simulink library "collection_of_goodies"  (R2018a)
settings: Solver=VariableStepAuto  StartTime=0.0  StopTime=10.0  RelTol=1e-3
undefined symbols (not defined in the file or in its folder): a1_T_CMG, a2_T_CMG, a3_T_CMG, AccLim, b1_T_CMG, b2_T_CMG, b3_T_CMG, c, CFthreshoff, CFthreshon, filt1d, filt1n, filt2d, filt2n, filts1n, filts2d, filts2n, fine, h, h_cos_cmg, h_init, h_sin_cmg, hdmax, hmax, I, I34, Id, Igm1d, Igm1n, IgmAAFd, init, invI, invId, Is, Isat, IsatSp, k1_obs, k2_obs, Kt, Kts, lam, Lgm, ls, lt, M34, Ngear, P0, pfd, pfn, q0, q_init, rc_ampl, rc_harm, rc_phase, Rgm, Smin, SmotDrag, spin_init, TachAAFd, TAU_ACS ... (+9)
libraries: mblibv1 x3, sharedutil x1, dspinverses x1, $bdroot x1
(part 2 of 3)

== system collection_of_goodies/Vector Math/3x3 cross ==
  v : Inport
  Constant1 : Constant  Value=0
  Constant2 : Constant  Value=0
  Constant3 : Constant  Value=0
  Demux : Demux  Outputs=3
  Gain : Gain  Gain=-1  SaturateOnIntegerOverflow=on  OutDataTypeStr=Inherit: Same as input  ParamDataTypeStr=Inherit: Same as input
  Gain1 : Gain  Gain=-1  SaturateOnIntegerOverflow=on  OutDataTypeStr=Inherit: Same as input  ParamDataTypeStr=Inherit: Same as input
  Gain2 : Gain  Gain=-1  SaturateOnIntegerOverflow=on  OutDataTypeStr=Inherit: Same as input  ParamDataTypeStr=Inherit: Same as input
  Matrix Concatenation : Concatenate  NumInputs=3  Mode=Multidimensional array  ConcatenateDimension=2
  Mux1 : Mux  Inputs=3
  Mux2 : Mux  Inputs=3
  Mux3 : Mux  Inputs=3
  vX : Outport
  wires:
  v/1 -> Demux/1
  Matrix Concatenation/1 -> vX/1
  Mux3/1 -> Matrix Concatenation/1
  Mux1/1 -> Matrix Concatenation/2
  Mux2/1 -> Matrix Concatenation/3
  Gain/1 -> Mux3/3
  Gain1/1 -> Mux1/1
  Gain2/1 -> Mux2/2
  Constant1/1 -> Mux3/1
  Constant2/1 -> Mux1/2
  Constant3/1 -> Mux2/3
  Demux/3 -> Mux3/2, Gain1/1
  Demux/2 -> Gain/1, Mux2/1
  Demux/1 -> Mux1/3, Gain2/1

== system collection_of_goodies/Vector Math/Cross ==
  A : Inport
  B : Inport  Port=2
  Mux4 : Mux  Inputs=3
  Product{,1..5} (6 alike) : Product  SaturateOnIntegerOverflow=on  InputSameDT=on  OutDataTypeStr=Inherit: Same as first input
  Sum : Sum  Inputs=+-  SaturateOnIntegerOverflow=on  InputSameDT=on  OutDataTypeStr=Inherit: Same as first input
  Sum1 : Sum  Inputs=+-  SaturateOnIntegerOverflow=on  InputSameDT=on  OutDataTypeStr=Inherit: Same as first input
  Sum2 : Sum  Inputs=+-  SaturateOnIntegerOverflow=on  InputSameDT=on  OutDataTypeStr=Inherit: Same as first input
  demux2 : Demux  Outputs=3
  demux3 : Demux  Outputs=3
  AxB : Outport  InitialOutput=0
  wires:
  Mux4/1 -> AxB/1
  Sum2/1 -> Mux4/3
  Sum1/1 -> Mux4/2
  Sum/1 -> Mux4/1
  Product5/1 -> Sum2/2
  Product4/1 -> Sum2/1
  Product3/1 -> Sum1/2
  Product2/1 -> Sum1/1
  Product1/1 -> Sum/2
  Product/1 -> Sum/1
  demux3/1 -> Product5/2, Product2/2
  demux2/2 -> Product5/1, Product/1
  demux3/2 -> Product4/2, Product1/2
  demux2/1 -> Product4/1, Product3/1
  demux3/3 -> Product3/2, Product/2
  demux2/3 -> Product2/1, Product1/1
  B/1 -> demux3/1
  A/1 -> demux2/1

== system collection_of_goodies/Vector Math/cross2 ==
  a : Inport
  b : Inport  Port=2
  Demux : Demux  Outputs=3
  Demux1 : Demux  Outputs=3
  Fcn : Fcn  Expr=-u(3)*u(5)+u(2)*u(6)
  Fcn1 : Fcn  Expr=u(3)*u(4)-u(1)*u(6)
  Fcn2 : Fcn  Expr=-u(2)*u(4)+u(1)*u(5)
  Mux : Mux  Inputs=6
  Mux1 : Mux  Inputs=3
  a x b : Outport
  wires:
  Mux/1 -> Fcn/1, Fcn1/1, Fcn2/1
  Mux1/1 -> a x b/1
  Fcn/1 -> Mux1/1
  Fcn1/1 -> Mux1/2
  Fcn2/1 -> Mux1/3
  Demux/1 -> Mux/1
  Demux/2 -> Mux/2
  Demux/3 -> Mux/3
  a/1 -> Demux/1
  Demux1/1 -> Mux/4
  Demux1/2 -> Mux/5
  Demux1/3 -> Mux/6
  b/1 -> Demux1/1

== system collection_of_goodies/Vector Math/norm ==
  v : Inport
  Dot Product : DotProduct  InputSameDT=on  OutDataTypeStr=Inherit: Inherit via internal rule
  Math Function : Math  Operator=sqrt  SaturateOnIntegerOverflow=on
  |v| : Outport
  wires:
  Math Function/1 -> |v|/1
  Dot Product/1 -> Math Function/1
  v/1 -> Dot Product/2, Dot Product/1

== system collection_of_goodies/Vector Math/normalize ==
  v : Inport
  Dot Product : DotProduct  InputSameDT=on  OutDataTypeStr=Inherit: Inherit via internal rule
  Math Function : Math  Operator=sqrt  SaturateOnIntegerOverflow=on
  Product : Product  Inputs=*/  SaturateOnIntegerOverflow=on  InputSameDT=on  OutDataTypeStr=Inherit: Same as first input
  v_hat : Outport
  wires:
  v/1 -> Dot Product/1, Dot Product/2, Product/1
  Dot Product/1 -> Math Function/1
  Math Function/1 -> Product/2
  Product/1 -> v_hat/1

== system collection_of_goodies/Vector Math/uncross ==
  v^x : Inport
  Demux : Demux  Outputs=9
  Mux : Mux  Inputs=3
  Reshape : Reshape
  Terminator{,1..5} (6 alike) : Terminator
  v : Outport
  wires:
  Mux/1 -> v/1
  v^x/1 -> Reshape/1
  Demux/1 -> Terminator/1
  Demux/5 -> Terminator1/1
  Demux/9 -> Terminator4/1
  Demux/8 -> Terminator5/1
  Demux/2 -> Mux/3
  Demux/4 -> Terminator2/1
  Demux/7 -> Mux/2
  Demux/3 -> Terminator3/1
  Demux/6 -> Mux/1
  Reshape/1 -> Demux/1

== system collection_of_goodies/Attitude Dynamics/AttitudeObserver/AttError ==
  q_meas : Inport  PortDimensions=4
  q_est : Inport  Port=2  PortDimensions=4
  Demux : Demux
  Gain : Gain  Gain=2  SaturateOnIntegerOverflow=on  OutDataTypeStr=Inherit: Same as input  ParamDataTypeStr=Inherit: Same as input
  Mux : Mux  Inputs=3
  Terminator : Terminator
  qconjMult : Subsystem
  att_err : Outport
  wires:
  q_est/1 -> qconjMult/1(q_cmd)
  q_meas/1 -> qconjMult/2(q_est)
  qconjMult/1(q_err) -> Demux/1
  Demux/1 -> Mux/1
  Demux/2 -> Mux/2
  Demux/3 -> Mux/3
  Mux/1 -> Gain/1
  Gain/1 -> att_err/1
  Demux/4 -> Terminator/1

== system collection_of_goodies/Attitude Dynamics/AttitudeObserver/q_normalize ==
  q_in : Inport  PortDimensions=4
  Dot Product : DotProduct  InputSameDT=on  OutDataTypeStr=Inherit: Inherit via internal rule
  Math Function : Math  Operator=sqrt  SaturateOnIntegerOverflow=on
  Product : Product  Inputs=*/  SaturateOnIntegerOverflow=on  InputSameDT=on  OutDataTypeStr=Inherit: Same as first input
  q_out : Outport
  wires:
  q_in/1 -> Dot Product/1, Dot Product/2, Product/1
  Dot Product/1 -> Math Function/1
  Math Function/1 -> Product/2
  Product/1 -> q_out/1

== system collection_of_goodies/Attitude Dynamics/AttitudeObserver/qderiv ==
  w : Inport
  q : Inport  Port=2
  Mux : Mux  Inputs=2
  Mux1 : Mux
  qd1 : Fcn  Expr=(u(7)*u(1)-u(6)*u(2)+u(5)*u(3))/2
  qd2 : Fcn  Expr=(u(6)*u(1)+u(7)*u(2)-u(4)*u(3))/2
  qd3 : Fcn  Expr=(-u(5)*u(1)+u(4)*u(2)+u(7)*u(3))/2
  qd4 : Fcn  Expr=(-u(4)*u(1)-u(5)*u(2)-u(6)*u(3))/2
  qd : Outport
  wires:
  w/1 -> Mux/1
  q/1 -> Mux/2
  Mux/1 -> qd3/1, qd4/1, qd1/1, qd2/1
  qd1/1 -> Mux1/1
  qd2/1 -> Mux1/2
  qd3/1 -> Mux1/3
  qd4/1 -> Mux1/4
  Mux1/1 -> qd/1

== system collection_of_goodies/Attitude Dynamics/CMG Array Model/Array_Steering ==
  note: This Jacobian is NOT designed
      | to be singularity free
  gimbal_rate : Inport  PortDimensions=6
  spin_rate_meas : Inport  Port=2  PortDimensions=6
  gim_ang_meas : Inport  Port=3  PortDimensions=6
  Compute_Amatrix : Subsystem
  Cosine : Trigonometry  Operator=cos
  Dot Product : DotProduct  InputSameDT=on  OutDataTypeStr=Inherit: Inherit via internal rule
  Dot Product1 : DotProduct  InputSameDT=on  OutDataTypeStr=Inherit: Inherit via internal rule
  Dot Product2 : DotProduct  InputSameDT=on  OutDataTypeStr=Inherit: Inherit via internal rule
  Mux : Mux  Inputs=3
  Product : Product  SaturateOnIntegerOverflow=on  InputSameDT=on  OutDataTypeStr=Inherit: Same as first input
  Product1 : Product  SaturateOnIntegerOverflow=on  InputSameDT=on  OutDataTypeStr=Inherit: Same as first input
  Product2 : Product  SaturateOnIntegerOverflow=on  InputSameDT=on  OutDataTypeStr=Inherit: Same as first input
  Sine : Trigonometry
  wheel_inertias : Constant  Value=wheel_inertias
  torque : Outport
  wires:
  Mux/1 -> torque/1
  Dot Product/1 -> Mux/1
  Dot Product2/1 -> Mux/3
  Dot Product1/1 -> Mux/2
  gimbal_rate/1 -> Dot Product2/2, Dot Product1/2, Dot Product/2
  Compute_Amatrix/3(Arow3) -> Dot Product2/1
  Compute_Amatrix/2(Arow2) -> Dot Product1/1
  Compute_Amatrix/1(Arow1) -> Dot Product/1
  Product2/1 -> Product1/1, Product/1
  wheel_inertias/1 -> Product2/1
  spin_rate_meas/1 -> Product2/2
  Cosine/1 -> Product1/2
  Sine/1 -> Product/2
  gim_ang_meas/1 -> Cosine/1, Sine/1
  Product1/1 -> Compute_Amatrix/2(cos_term)
  Product/1 -> Compute_Amatrix/1(sin_term)

== system collection_of_goodies/Attitude Dynamics/CMG Array Model/ComputeCMGMomentum ==
  spin_rate_meas : Inport  PortDimensions=6
  gim_ang_meas : Inport  Port=2  PortDimensions=6
  Cosine : Trigonometry  Operator=cos
  Product : Product  SaturateOnIntegerOverflow=on  InputSameDT=on  OutDataTypeStr=Inherit: Same as first input
  Product1 : Product  SaturateOnIntegerOverflow=on  InputSameDT=on  OutDataTypeStr=Inherit: Same as first input
  Product2 : Product  SaturateOnIntegerOverflow=on  InputSameDT=on  OutDataTypeStr=Inherit: Same as first input
  Sine : Trigonometry
  Sum : Sum  SaturateOnIntegerOverflow=on  InputSameDT=on  OutDataTypeStr=Inherit: Same as first input
  h_cos : Gain  Gain=h_cos_cmg  Multiplication=Matrix(K*u)  SaturateOnIntegerOverflow=on  OutDataTypeStr=Inherit: Same as input  ParamDataTypeStr=Inherit: Same as input
  h_sin : Gain  Gain=h_sin_cmg  Multiplication=Matrix(K*u)  SaturateOnIntegerOverflow=on  OutDataTypeStr=Inherit: Same as input  ParamDataTypeStr=Inherit: Same as input
  wheel_inertias : Constant  Value=wheel_inertias
  H_cmg : Outport
  wires:
  gim_ang_meas/1 -> Sine/1, Cosine/1
  Sine/1 -> Product/2
  Cosine/1 -> Product1/2
  h_sin/1 -> Sum/1
  h_cos/1 -> Sum/2
  spin_rate_meas/1 -> Product2/2
  wheel_inertias/1 -> Product2/1
  Product2/1 -> Product/1, Product1/1
  Sum/1 -> H_cmg/1
  Product1/1 -> h_cos/1
  Product/1 -> h_sin/1

== system collection_of_goodies/Attitude Dynamics/CMG Array Model/WxH (gyroscopic torque) ==
  v1 : Inport
  v2 : Inport  Port=2
  Cross1 : Fcn  Expr=-u(3)*u(5)+u(2)*u(6)
  Cross2 : Fcn  Expr=u(3)*u(4)-u(1)*u(6)
  Cross3 : Fcn  Expr=-u(2)*u(4)+u(1)*u(5)
  Mux : Mux  Inputs=2
  Mux1 : Mux  Inputs=3
  v1xv2 : Outport
  wires:
  v1/1 -> Mux/1
  v2/1 -> Mux/2
  Mux/1 -> Cross1/1, Cross2/1, Cross3/1
  Cross2/1 -> Mux1/2
  Cross1/1 -> Mux1/1
  Cross3/1 -> Mux1/3
  Mux1/1 -> v1xv2/1

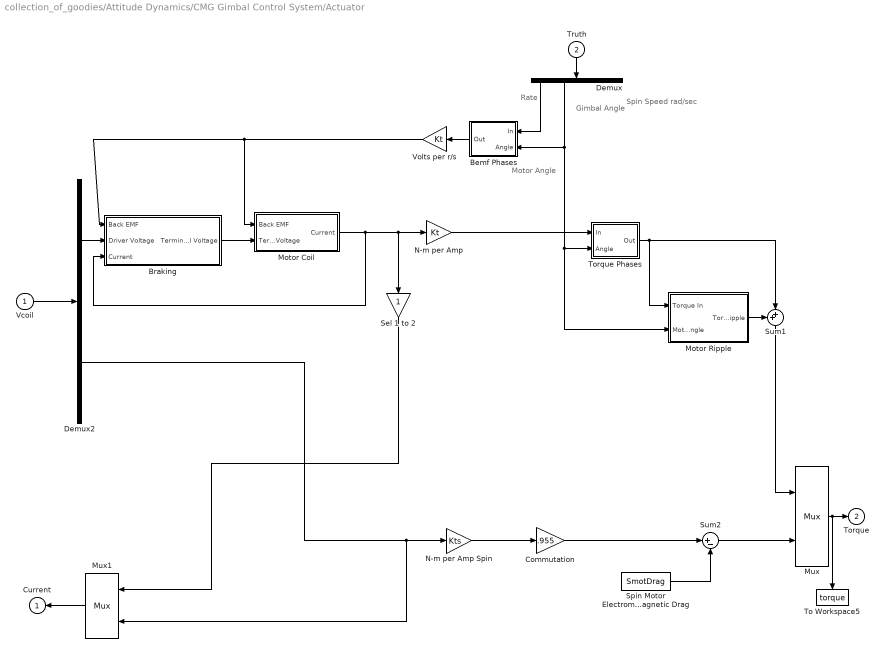
== system collection_of_goodies/Attitude Dynamics/CMG Gimbal Control System/Actuator ==
  note: Rate
  note: Motor Angle
  note: Spin
      | Speed
      | rad/sec
  note: Gimbal
      | Angle
  Vcoil : Inport
  Truth : Inport  Port=2
  Bemf Phases : Subsystem
  Braking : Subsystem
  Commutation : Gain  Gain=.955  SaturateOnIntegerOverflow=on  OutDataTypeStr=Inherit: Same as input  ParamDataTypeStr=Inherit: Same as input
  Demux : Demux
  Demux2 : Demux  Outputs=[2 1]
  Motor Coil : Subsystem
  Motor Ripple : Subsystem
  Mux : Mux  Inputs=2
  Mux1 : Mux  Inputs=[2 1]
  N-m per Amp : Gain  Gain=Kt  SaturateOnIntegerOverflow=on  OutDataTypeStr=Inherit: Same as input  ParamDataTypeStr=Inherit: Same as input
  N-m per Amp Spin : Gain  Gain=Kts  SaturateOnIntegerOverflow=on  OutDataTypeStr=Inherit: Same as input  ParamDataTypeStr=Inherit: Same as input
  Sel 1 to 2 : Gain  SaturateOnIntegerOverflow=on  OutDataTypeStr=Inherit: Same as input  ParamDataTypeStr=Inherit: Same as input
  Spin Motor Electromagnetic Drag : Constant  Value=SmotDrag
  Sum1 : Sum  Inputs=++|  SaturateOnIntegerOverflow=on  InputSameDT=on  OutDataTypeStr=Inherit: Same as first input
  Sum2 : Sum  Inputs=|+-  SaturateOnIntegerOverflow=on  InputSameDT=on  OutDataTypeStr=Inherit: Same as first input
  To Workspace5 : ToWorkspace  VariableName=torque  SampleTime=-1
  Torque Phases : Subsystem
  Volts per r/s : Gain  Gain=Kt  SaturateOnIntegerOverflow=on  OutDataTypeStr=Inherit: Same as input  ParamDataTypeStr=Inherit: Same as input
  Current : Outport  InitialOutput=0
  Torque : Outport  Port=2  InitialOutput=0
  wires:
  Mux1/1 -> Current/1
  Bemf Phases/1(Out) -> Volts per r/s/1
  N-m per Amp/1 -> Torque Phases/1(In)
  Sel 1 to 2/1 -> Mux1/1
  Spin Motor Electromagnetic Drag/1 -> Sum2/2
  Sum2/1 -> Mux/2
  Mux/1 -> Torque/1, To Workspace5/1
  Demux/1 -> Bemf Phases/1(In)
  Motor Ripple/1(Torque Ripple) -> Sum1/1
  Sum1/1 -> Mux/1
  Truth/1 -> Demux/1
  Demux/2 -> Bemf Phases/2(Angle), Torque Phases/2(Angle), Motor Ripple/2(Motor Angle)
  Torque Phases/1(Out) -> Motor Ripple/1(Torque In), Sum1/2
  N-m per Amp Spin/1 -> Commutation/1
  Commutation/1 -> Sum2/1
  Braking/1(Terminal Voltage) -> Motor Coil/2(Terminal Voltage)
  Motor Coil/1(Current) -> N-m per Amp/1, Sel 1 to 2/1, Braking/3(Current)
  Volts per r/s/1 -> Motor Coil/1(Back EMF), Braking/1(Back EMF)
  Demux2/2 -> N-m per Amp Spin/1, Mux1/2
  Demux2/1 -> Braking/2(Driver Voltage)
  Vcoil/1 -> Demux2/1

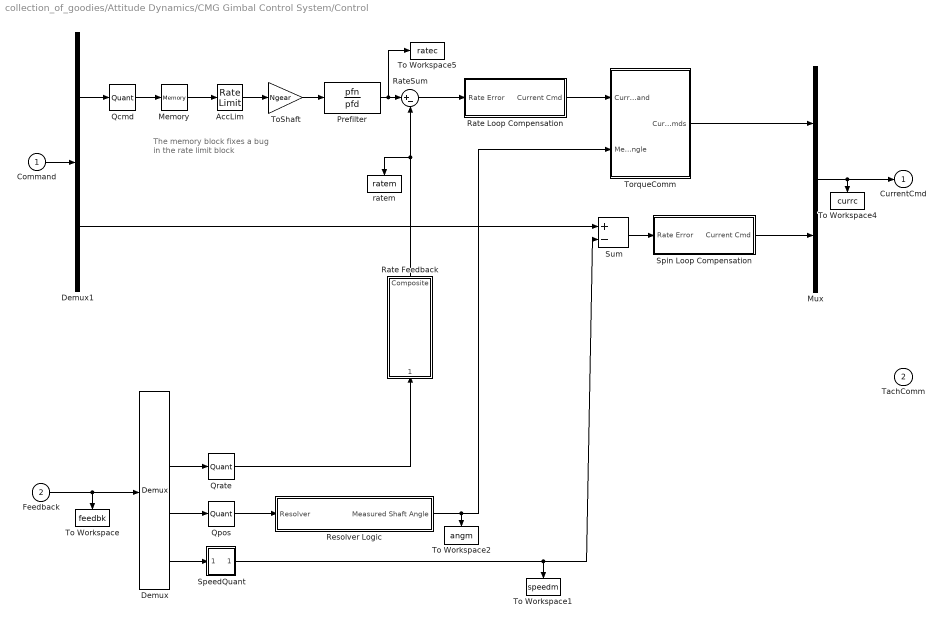
== system collection_of_goodies/Attitude Dynamics/CMG Gimbal Control System/Control ==
  note: The memory block fixes
      | a bug in the rate limit block
  Command : Inport  PortDimensions=2
  Feedback : Inport  Port=2
  AccLim : RateLimiter  RisingSlewLimit=AccLim  FallingSlewLimit=-AccLim
  Demux : Demux  Outputs=[3 2 4 1]
  Demux1 : Demux  Outputs=2
  Memory : Memory
  Mux : Mux  Inputs=[2 1]
  Prefilter : TransferFcn  Numerator=pfn  Denominator=pfd
  Qcmd : Quantizer  QuantizationInterval=Qcmd
  Qpos : Quantizer  QuantizationInterval=Qpos
  Qrate : Quantizer  QuantizationInterval=Qrate
  Rate Feedback : Subsystem
  Rate Loop Compensation : Subsystem
  RateSum : Sum  Inputs=|+-  SaturateOnIntegerOverflow=on  InputSameDT=on  OutDataTypeStr=Inherit: Same as first input
  Resolver Logic : Subsystem
  SpeedQuant : Subsystem
  Spin Loop Compensation : Subsystem
  Sum : Sum  Inputs=+-  SaturateOnIntegerOverflow=on  InputSameDT=on  OutDataTypeStr=Inherit: Same as first input
  To Workspace : ToWorkspace  VariableName=feedbk  SampleTime=-1
  To Workspace1 : ToWorkspace  VariableName=speedm  SampleTime=-1
  To Workspace2 : ToWorkspace  VariableName=angm  SampleTime=-1
  To Workspace4 : ToWorkspace  VariableName=currc  SampleTime=-1
  To Workspace5 : ToWorkspace  VariableName=ratec  SampleTime=-1
  ToShaft : Gain  Gain=Ngear  OutDataTypeStr=Inherit: Same as input  ParamDataTypeStr=Inherit: Same as input
  TorqueComm : Subsystem
  ratem : ToWorkspace  VariableName=ratem  SampleTime=-1
  CurrentCmd : Outport  InitialOutput=0
  TachComm : Outport  Port=2  InitialOutput=0
  wires:
  Demux/2 -> Qrate/1
  Demux/3 -> Qpos/1
  Qpos/1 -> Resolver Logic/1(Resolver)
  Demux/4 -> SpeedQuant/1(In)
  SpeedQuant/1(Out) -> Sum/2, To Workspace1/1
  Resolver Logic/1(Measured Shaft Angle) -> TorqueComm/2(Meas Shaft Angle), To Workspace2/1
  Feedback/1 -> Demux/1, To Workspace/1
  Command/1 -> Demux1/1
  Qrate/1 -> Rate Feedback/1(Coarse/Fine)
  Qcmd/1 -> Memory/1
  AccLim/1 -> ToShaft/1
  Demux1/1 -> Qcmd/1
  Memory/1 -> AccLim/1
  TorqueComm/1(Current Cmds) -> Mux/1
  ToShaft/1 -> Prefilter/1
  Prefilter/1 -> RateSum/1, To Workspace5/1
  Sum/1 -> Spin Loop Compensation/1(Rate Error)
  Spin Loop Compensation/1(Current Cmd) -> Mux/2
  Demux1/2 -> Sum/1
  Mux/1 -> CurrentCmd/1, To Workspace4/1
  Rate Feedback/1(Composite) -> RateSum/2, ratem/1
  RateSum/1 -> Rate Loop Compensation/1(Rate Error)
  Rate Loop Compensation/1(Current Cmd) -> TorqueComm/1(Current Command)

== system collection_of_goodies/Attitude Dynamics/CMG Gimbal Control System/Drive ==
  Current : Inport
  CurrentCmd : Inport  Port=2
  Current Loop 1 : Subsystem
  Current Loop 2 : Subsystem
  Demux1 : Demux  Outputs=3
  Demux2 : Demux  Outputs=3
  Mux : Mux  Inputs=3
  Mux1 : Mux  Inputs=3
  To Workspace4 : ToWorkspace  VariableName=curr  SampleTime=-1
  To Workspace5 : ToWorkspace  VariableName=vcoil  SampleTime=-1
  Vcoil : Outport  InitialOutput=0
  CurSense : Outport  Port=2  InitialOutput=0
  wires:
  CurrentCmd/1 -> Demux1/1
  Demux1/3 -> Mux/3
  Mux1/1 -> CurSense/1
  Demux2/3 -> Mux1/3
  Demux1/1 -> Current Loop 1/1(CurrentCmd)
  Demux1/2 -> Current Loop 2/1(CurrentCmd)
  Demux2/1 -> Current Loop 1/2(Current)
  Demux2/2 -> Current Loop 2/2(Current)
  Current Loop 1/1(Vanalog) -> Mux/1
  Current Loop 2/1(Vanalog) -> Mux/2
  Current Loop 1/2(CurSense) -> Mux1/1
  Current Loop 2/2(CurSense) -> Mux1/2
  Current/1 -> Demux2/1, To Workspace4/1
  Mux/1 -> Vcoil/1, To Workspace5/1

== system collection_of_goodies/Attitude Dynamics/CMG Gimbal Control System/Sensor ==
  note: Motor Angle
  note: Gimbal Angle
  note: Motor
      | Rate
  TachComm : Inport
  CurSense : Inport  Port=2
  Truth : Inport  Port=3
  AAF : TransferFcn  Denominator=TachAAFd
  Demux : Demux
  Fine Gain : Gain  Gain=fine  SaturateOnIntegerOverflow=on  OutDataTypeStr=Inherit: Same as input  ParamDataTypeStr=Inherit: Same as input
  Mux : Mux  Inputs=[3 1 1 4 1]
  Resolvers : Subsystem
  Tach Phases : Subsystem
  Tach Ripple : Subsystem
  Tachometer : Sum  Inputs=|++  SaturateOnIntegerOverflow=on  InputSameDT=on  OutDataTypeStr=Inherit: Same as first input
  Sensor : Outport  InitialOutput=0
  wires:
  Mux/1 -> Sensor/1
  Tach Phases/1(Meas Rate) -> AAF/1
  Fine Gain/1 -> Mux/3
  Tachometer/1 -> Tach Phases/2(Rate)
  CurSense/1 -> Mux/1
  TachComm/1 -> Tach Phases/1(TachComm)
  AAF/1 -> Mux/2, Fine Gain/1
  Demux/2 -> Tach Ripple/2(Motor Angle), Tach Phases/3(Truth Angle), Resolvers/1(Truth Angle)
  Resolvers/1(Resolver Out) -> Mux/4
  Demux/1 -> Tachometer/1, Tach Ripple/1(Rate In)
  Tach Ripple/1(Tach Ripple) -> Tachometer/2
  Truth/1 -> Demux/1
  Demux/4 -> Mux/5

== system collection_of_goodies/Attitude Dynamics/Kane Damper wbn is inertial body rate in body axes apply (-Tdamp) to rigid body/Cross1 ==
  A : Inport
  B : Inport  Port=2
  Mux4 : Mux  Inputs=3
  Product{,1..5} (6 alike) : Product  SaturateOnIntegerOverflow=on  InputSameDT=on  OutDataTypeStr=Inherit: Same as first input
  Sum : Sum  Inputs=+-  SaturateOnIntegerOverflow=on  InputSameDT=on  OutDataTypeStr=Inherit: Same as first input
  Sum1 : Sum  Inputs=+-  SaturateOnIntegerOverflow=on  InputSameDT=on  OutDataTypeStr=Inherit: Same as first input
  Sum2 : Sum  Inputs=+-  SaturateOnIntegerOverflow=on  InputSameDT=on  OutDataTypeStr=Inherit: Same as first input
  demux2 : Demux  Outputs=3
  demux3 : Demux  Outputs=3
  AxB : Outport  InitialOutput=0
  wires:
  Mux4/1 -> AxB/1
  Sum2/1 -> Mux4/3
  Sum1/1 -> Mux4/2
  Sum/1 -> Mux4/1
  Product5/1 -> Sum2/2
  Product4/1 -> Sum2/1
  Product3/1 -> Sum1/2
  Product2/1 -> Sum1/1
  Product1/1 -> Sum/2
  Product/1 -> Sum/1
  demux3/1 -> Product5/2, Product2/2
  demux2/2 -> Product5/1, Product/1
  demux3/2 -> Product4/2, Product1/2
  demux2/1 -> Product4/1, Product3/1
  demux3/3 -> Product3/2, Product/2
  demux2/3 -> Product2/1, Product1/1
  B/1 -> demux3/1
  A/1 -> demux2/1

== system collection_of_goodies/Attitude Dynamics/Propagate Attitude via DCM (not as nice as the quaternion method)/(a*phi)^X ==
  In1 : Inport
  3x3 : Reshape  OutputDimensionality=Customize  OutputDimensions=[3,3]
  Demux : Demux  Outputs=3
  Gain : Gain  Gain=-1  SaturateOnIntegerOverflow=on  OutDataTypeStr=Inherit: Same as input  ParamDataTypeStr=Inherit: Same as input
  Gain1 : Gain  Gain=-1  SaturateOnIntegerOverflow=on  OutDataTypeStr=Inherit: Same as input  ParamDataTypeStr=Inherit: Same as input
  Gain2 : Gain  Gain=-1  SaturateOnIntegerOverflow=on  OutDataTypeStr=Inherit: Same as input  ParamDataTypeStr=Inherit: Same as input
  Mux : Mux  Inputs=9
  "diag 0 " : Constant  Value=0
  Out1 : Outport
  wires:
  In1/1 -> Demux/1
  3x3/1 -> Out1/1
  "diag 0 "/1 -> Mux/1, Mux/5, Mux/9
  Mux/1 -> 3x3/1
  Demux/3 -> Mux/2, Gain1/1
  Gain/1 -> Mux/3
  Demux/2 -> Gain/1, Mux/7
  Gain1/1 -> Mux/4
  Demux/1 -> Mux/6, Gain2/1
  Gain2/1 -> Mux/8

== system collection_of_goodies/Attitude Dynamics/Propagate Attitude via Quaternion/q_normalize ==
  q_in : Inport  PortDimensions=4
  Dot Product : DotProduct  InputSameDT=on  OutDataTypeStr=Inherit: Inherit via internal rule
  Math Function : Math  Operator=sqrt  SaturateOnIntegerOverflow=on
  Product : Product  Inputs=*/  SaturateOnIntegerOverflow=on  InputSameDT=on  OutDataTypeStr=Inherit: Same as first input
  q_out : Outport
  wires:
  q_in/1 -> Dot Product/1, Dot Product/2, Product/1
  Dot Product/1 -> Math Function/1
  Math Function/1 -> Product/2
  Product/1 -> q_out/1

== system collection_of_goodies/Attitude Dynamics/Propagate Attitude via Quaternion/quat_multiply ==
  q_bc : Inport
  q_ab : Inport  Port=2
  Mux : Mux  Inputs=2
  Mux1 : Mux
  qerr1 : Fcn  Expr=u(4)*u(5)+u(3)*u(6)-u(2)*u(7)+u(1)*u(8)
  qerr2 : Fcn  Expr=-u(3)*u(5)+u(4)*u(6)+u(1)*u(7)+u(2)*u(8)
  qerr3 : Fcn  Expr=u(2)*u(5)-u(1)*u(6)+u(4)*u(7)+u(3)*u(8)
  qerr4 : Fcn  Expr=-u(1)*u(5)-u(2)*u(6)-u(3)*u(7)+u(4)*u(8)
  q_ac : Outport
  wires:
  Mux1/1 -> q_ac/1
  qerr4/1 -> Mux1/4
  qerr3/1 -> Mux1/3
  qerr2/1 -> Mux1/2
  qerr1/1 -> Mux1/1
  Mux/1 -> qerr4/1, qerr3/1, qerr2/1, qerr1/1
  q_ab/1 -> Mux/2
  q_bc/1 -> Mux/1

== system collection_of_goodies/Attitude Dynamics/Quaternion Integration/q_normalize ==
  q_in : Inport  PortDimensions=4
  Dot Product : DotProduct  InputSameDT=on  OutDataTypeStr=Inherit: Inherit via internal rule
  Math Function : Math  Operator=sqrt  SaturateOnIntegerOverflow=on
  Product : Product  Inputs=*/  SaturateOnIntegerOverflow=on  InputSameDT=on  OutDataTypeStr=Inherit: Same as first input
  q_out : Outport
  wires:
  q_in/1 -> Dot Product/1, Dot Product/2, Product/1
  Dot Product/1 -> Math Function/1
  Math Function/1 -> Product/2
  Product/1 -> q_out/1

== system collection_of_goodies/Attitude Dynamics/Quaternion Integration/qderiv ==
  w : Inport
  q : Inport  Port=2
  Mux : Mux  Inputs=2
  Mux1 : Mux
  qd1 : Fcn  Expr=(u(7)*u(1)-u(6)*u(2)+u(5)*u(3))/2
  qd2 : Fcn  Expr=(u(6)*u(1)+u(7)*u(2)-u(4)*u(3))/2
  qd3 : Fcn  Expr=(-u(5)*u(1)+u(4)*u(2)+u(7)*u(3))/2
  qd4 : Fcn  Expr=(-u(4)*u(1)-u(5)*u(2)-u(6)*u(3))/2
  qd : Outport
  wires:
  w/1 -> Mux/1
  q/1 -> Mux/2
  Mux/1 -> qd1/1, qd2/1, qd3/1, qd4/1
  qd1/1 -> Mux1/1
  qd2/1 -> Mux1/2
  qd3/1 -> Mux1/3
  qd4/1 -> Mux1/4
  Mux1/1 -> qd/1

== system collection_of_goodies/Attitude Dynamics/Rigid Body with Momentum Actuators and energy dissipation/Cross ==
  A : Inport
  B : Inport  Port=2
  Mux4 : Mux  Inputs=3
  Product{,1..5} (6 alike) : Product  SaturateOnIntegerOverflow=on  InputSameDT=on  OutDataTypeStr=Inherit: Same as first input
  Sum : Sum  Inputs=+-  SaturateOnIntegerOverflow=on  InputSameDT=on  OutDataTypeStr=Inherit: Same as first input
  Sum1 : Sum  Inputs=+-  SaturateOnIntegerOverflow=on  InputSameDT=on  OutDataTypeStr=Inherit: Same as first input
  Sum2 : Sum  Inputs=+-  SaturateOnIntegerOverflow=on  InputSameDT=on  OutDataTypeStr=Inherit: Same as first input
  demux2 : Demux  Outputs=3
  demux3 : Demux  Outputs=3
  AxB : Outport  InitialOutput=0
  wires:
  Mux4/1 -> AxB/1
  Sum2/1 -> Mux4/3
  Sum1/1 -> Mux4/2
  Sum/1 -> Mux4/1
  Product5/1 -> Sum2/2
  Product4/1 -> Sum2/1
  Product3/1 -> Sum1/2
  Product2/1 -> Sum1/1
  Product1/1 -> Sum/2
  Product/1 -> Sum/1
  demux3/1 -> Product5/2, Product2/2
  demux2/2 -> Product5/1, Product/1
  demux3/2 -> Product4/2, Product1/2
  demux2/1 -> Product4/1, Product3/1
  demux3/3 -> Product3/2, Product/2
  demux2/3 -> Product2/1, Product1/1
  B/1 -> demux3/1
  A/1 -> demux2/1

== system collection_of_goodies/Attitude Dynamics/Rigid Body with Momentum Actuators and energy dissipation/Cross1 ==
  A : Inport
  B : Inport  Port=2
  Mux4 : Mux  Inputs=3
  Product{,1..5} (6 alike) : Product  SaturateOnIntegerOverflow=on  InputSameDT=on  OutDataTypeStr=Inherit: Same as first input
  Sum : Sum  Inputs=+-  SaturateOnIntegerOverflow=on  InputSameDT=on  OutDataTypeStr=Inherit: Same as first input
  Sum1 : Sum  Inputs=+-  SaturateOnIntegerOverflow=on  InputSameDT=on  OutDataTypeStr=Inherit: Same as first input
  Sum2 : Sum  Inputs=+-  SaturateOnIntegerOverflow=on  InputSameDT=on  OutDataTypeStr=Inherit: Same as first input
  demux2 : Demux  Outputs=3
  demux3 : Demux  Outputs=3
  AxB : Outport  InitialOutput=0
  wires:
  Mux4/1 -> AxB/1
  Sum2/1 -> Mux4/3
  Sum1/1 -> Mux4/2
  Sum/1 -> Mux4/1
  Product5/1 -> Sum2/2
  Product4/1 -> Sum2/1
  Product3/1 -> Sum1/2
  Product2/1 -> Sum1/1
  Product1/1 -> Sum/2
  Product/1 -> Sum/1
  demux3/1 -> Product5/2, Product2/2
  demux2/2 -> Product5/1, Product/1
  demux3/2 -> Product4/2, Product1/2
  demux2/1 -> Product4/1, Product3/1
  demux3/3 -> Product3/2, Product/2
  demux2/3 -> Product2/1, Product1/1
  B/1 -> demux3/1
  A/1 -> demux2/1

== system collection_of_goodies/Attitude Dynamics/Rigid Body with Momentum Actuators and energy dissipation/Quaternion Integration ==
  w_Body : Inport
  Integrator1 : Integrator  InitialCondition=q_init
  q_normalize : Subsystem
  qderiv : Subsystem
  q_I_Body : Outport
  wires:
  qderiv/1(qd) -> Integrator1/1
  Integrator1/1 -> q_normalize/1(q_in)
  q_normalize/1(q_out) -> q_I_Body/1, qderiv/2(q)
  w_Body/1 -> qderiv/1(w)

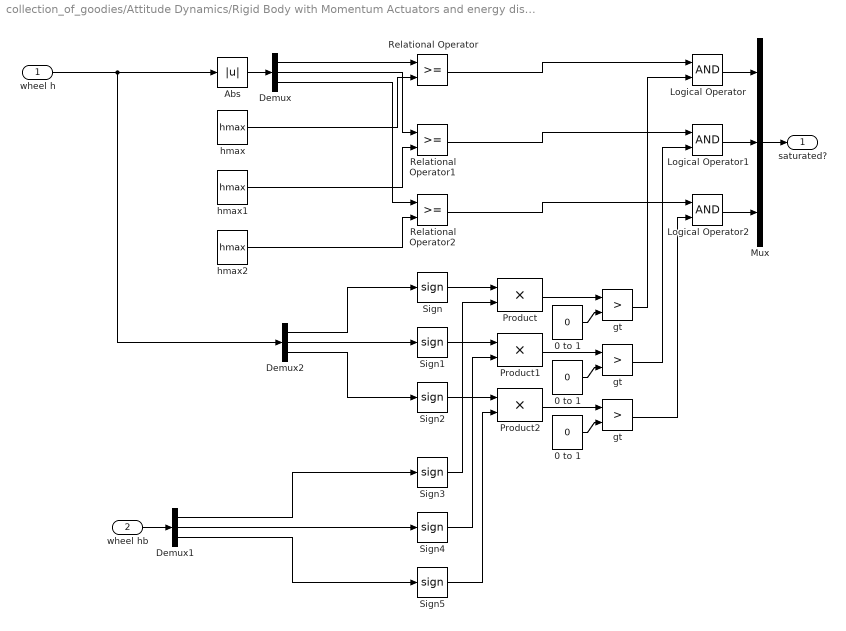
== system collection_of_goodies/Attitude Dynamics/Rigid Body with Momentum Actuators and energy dissipation/max rate check ==
  wheel h : Inport
  wheel hb : Inport  Port=2
  0 to 1 : Constant  Value=0  VectorParams1D=off
  "0 to 1 " : Constant  Value=0  VectorParams1D=off
  "0 to 1  " : Constant  Value=0  VectorParams1D=off
  Abs : Abs  SaturateOnIntegerOverflow=on
  Demux : Demux  Outputs=3
  Demux1 : Demux  Outputs=3
  Demux2 : Demux  Outputs=3
  Logical Operator : Logic
  Logical Operator1 : Logic
  Logical Operator2 : Logic
  Mux : Mux  Inputs=3
  Product : Product  SaturateOnIntegerOverflow=on  InputSameDT=on  OutDataTypeStr=Inherit: Same as first input
  Product1 : Product  SaturateOnIntegerOverflow=on  InputSameDT=on  OutDataTypeStr=Inherit: Same as first input
  Product2 : Product  SaturateOnIntegerOverflow=on  InputSameDT=on  OutDataTypeStr=Inherit: Same as first input
  Relational Operator : RelationalOperator  RndMeth=Nearest  InputSameDT=on
  Relational Operator1 : RelationalOperator  RndMeth=Nearest  InputSameDT=on
  Relational Operator2 : RelationalOperator  RndMeth=Nearest  InputSameDT=on
  Sign{,1..5} (6 alike) : Signum
  gt : RelationalOperator  Operator=>  RndMeth=Nearest  InputSameDT=on
  "gt " : RelationalOperator  Operator=>  RndMeth=Nearest  InputSameDT=on
  "gt  " : RelationalOperator  Operator=>  RndMeth=Nearest  InputSameDT=on
  hmax : Constant  Value=hmax  VectorParams1D=off
  hmax1 : Constant  Value=hmax  VectorParams1D=off
  hmax2 : Constant  Value=hmax  VectorParams1D=off
  saturated? : Outport
  wires:
  Abs/1 -> Demux/1
  Demux/1 -> Relational Operator/1
  Demux/2 -> Relational Operator1/1
  Demux/3 -> Relational Operator2/1
  hmax/1 -> Relational Operator/2
  hmax1/1 -> Relational Operator1/2
  hmax2/1 -> Relational Operator2/2
  wheel h/1 -> Abs/1, Demux2/1
  Mux/1 -> saturated?/1
  wheel hb/1 -> Demux1/1
  Demux1/1 -> Sign3/1
  Demux1/2 -> Sign4/1
  Demux1/3 -> Sign5/1
  Sign/1 -> Product/1
  Sign3/1 -> Product/2
  Sign1/1 -> Product1/1
  Sign4/1 -> Product1/2
  Sign2/1 -> Product2/1
  Sign5/1 -> Product2/2
  0 to 1/1 -> gt/2
  Product/1 -> gt/1
  "0 to 1 "/1 -> "gt "/2
  Product1/1 -> "gt "/1
  "0 to 1  "/1 -> "gt  "/2
  Product2/1 -> "gt  "/1
  Logical Operator/1 -> Mux/1
  Logical Operator1/1 -> Mux/2
  Logical Operator2/1 -> Mux/3
  Relational Operator/1 -> Logical Operator/1
  Relational Operator1/1 -> Logical Operator1/1
  Relational Operator2/1 -> Logical Operator2/1
  gt/1 -> Logical Operator/2
  "gt "/1 -> Logical Operator1/2
  "gt  "/1 -> Logical Operator2/2
  Demux2/1 -> Sign/1
  Demux2/2 -> Sign1/1
  Demux2/3 -> Sign2/1

== system collection_of_goodies/Attitude Dynamics/rigid body/Cross1 ==
  A : Inport  PortDimensions=3
  B : Inport  Port=2  PortDimensions=3
  Mux4 : Mux  Inputs=3
  Product{,1..5} (6 alike) : Product  SaturateOnIntegerOverflow=on  InputSameDT=on  OutDataTypeStr=Inherit: Same as first input
  Sum : Sum  Inputs=+-  SaturateOnIntegerOverflow=on  InputSameDT=on  OutDataTypeStr=Inherit: Same as first input
  Sum1 : Sum  Inputs=+-  SaturateOnIntegerOverflow=on  InputSameDT=on  OutDataTypeStr=Inherit: Same as first input
  Sum2 : Sum  Inputs=+-  SaturateOnIntegerOverflow=on  InputSameDT=on  OutDataTypeStr=Inherit: Same as first input
  demux2 : Demux  Outputs=3
  demux3 : Demux  Outputs=3
  AxB : Outport  InitialOutput=0
  wires:
  Mux4/1 -> AxB/1
  Sum2/1 -> Mux4/3
  Sum1/1 -> Mux4/2
  Sum/1 -> Mux4/1
  Product5/1 -> Sum2/2
  Product4/1 -> Sum2/1
  Product3/1 -> Sum1/2
  Product2/1 -> Sum1/1
  Product1/1 -> Sum/2
  Product/1 -> Sum/1
  demux3/1 -> Product5/2, Product2/2
  demux2/2 -> Product5/1, Product/1
  demux3/2 -> Product4/2, Product1/2
  demux2/1 -> Product4/1, Product3/1
  demux3/3 -> Product3/2, Product/2
  demux2/3 -> Product2/1, Product1/1
  B/1 -> demux3/1
  A/1 -> demux2/1

== system collection_of_goodies/Attitude Math/AttError/qconjMult ==
  q_cmd : Inport
  q_est : Inport  Port=2
  Mux : Mux  Inputs=2
  Mux1 : Mux
  qerr1 : Fcn  Expr=-u(4)*u(5)-u(3)*u(6)+u(2)*u(7)+u(1)*u(8)
  qerr2 : Fcn  Expr=u(3)*u(5)-u(4)*u(6)-u(1)*u(7)+u(2)*u(8)
  qerr3 : Fcn  Expr=-u(2)*u(5)+u(1)*u(6)-u(4)*u(7)+u(3)*u(8)
  qerr4 : Fcn  Expr=u(1)*u(5)+u(2)*u(6)+u(3)*u(7)+u(4)*u(8)
  q_err : Outport
  wires:
  q_cmd/1 -> Mux/1
  q_est/1 -> Mux/2
  Mux/1 -> qerr1/1, qerr2/1, qerr3/1, qerr4/1
  qerr1/1 -> Mux1/1
  qerr2/1 -> Mux1/2
  qerr3/1 -> Mux1/3
  qerr4/1 -> Mux1/4
  Mux1/1 -> q_err/1

== system collection_of_goodies/Attitude Math/attitude error as axis//angle/axis unit vector ==
  ax_in : Inport
  Constant : Constant  Value=1e-10
  Dot Product : DotProduct  InputSameDT=on  OutDataTypeStr=Inherit: Inherit via internal rule
  Math Function : Math  Operator=sqrt  SaturateOnIntegerOverflow=on
  Product : Product  Inputs=*/  SaturateOnIntegerOverflow=on  InputSameDT=on  OutDataTypeStr=Inherit: Same as first input
  Switch : Switch  Threshold=1e-10  SaturateOnIntegerOverflow=on  InputSameDT=on
  ax_out : Outport
  wires:
  ax_in/1 -> Dot Product/1, Dot Product/2, Product/1
  Dot Product/1 -> Math Function/1
  Math Function/1 -> Switch/2, Switch/1
  Constant/1 -> Switch/3
  Product/1 -> ax_out/1
  Switch/1 -> Product/2

== system collection_of_goodies/Attitude Math/attitude error as axis//angle/q_normalize ==
  q_in : Inport  PortDimensions=4
  Dot Product : DotProduct  InputSameDT=on  OutDataTypeStr=Inherit: Inherit via internal rule
  Math Function : Math  Operator=sqrt  SaturateOnIntegerOverflow=on
  Product : Product  Inputs=*/  SaturateOnIntegerOverflow=on  InputSameDT=on  OutDataTypeStr=Inherit: Same as first input
  q_out : Outport
  wires:
  q_in/1 -> Dot Product/1, Dot Product/2, Product/1
  Dot Product/1 -> Math Function/1
  Math Function/1 -> Product/2
  Product/1 -> q_out/1

== system collection_of_goodies/Attitude Math/attitude error as axis//angle/q_normalize1 ==
  q_in : Inport  PortDimensions=4
  Dot Product : DotProduct  InputSameDT=on  OutDataTypeStr=Inherit: Inherit via internal rule
  Math Function : Math  Operator=sqrt  SaturateOnIntegerOverflow=on
  Product : Product  Inputs=*/  SaturateOnIntegerOverflow=on  InputSameDT=on  OutDataTypeStr=Inherit: Same as first input
  q_out : Outport
  wires:
  q_in/1 -> Dot Product/1, Dot Product/2, Product/1
  Dot Product/1 -> Math Function/1
  Math Function/1 -> Product/2
  Product/1 -> q_out/1

== system collection_of_goodies/Attitude Math/attitude error as axis//angle/q_normalize2 ==
  q_in : Inport  PortDimensions=4
  Dot Product : DotProduct  InputSameDT=on  OutDataTypeStr=Inherit: Inherit via internal rule
  Math Function : Math  Operator=sqrt  SaturateOnIntegerOverflow=on
  Product : Product  Inputs=*/  SaturateOnIntegerOverflow=on  InputSameDT=on  OutDataTypeStr=Inherit: Same as first input
  q_out : Outport
  wires:
  q_in/1 -> Dot Product/1, Dot Product/2, Product/1
  Dot Product/1 -> Math Function/1
  Math Function/1 -> Product/2
  Product/1 -> q_out/1

== system collection_of_goodies/Attitude Math/attitude error as axis//angle/relative_quat1 ==
  q_bc : Inport
  q_ab : Inport  Port=2
  Mux : Mux  Inputs=2
  Mux1 : Mux
  qerr1 : Fcn  Expr=u(4)*u(5)+u(3)*u(6)-u(2)*u(7)+u(1)*u(8)
  qerr2 : Fcn  Expr=-u(3)*u(5)+u(4)*u(6)+u(1)*u(7)+u(2)*u(8)
  qerr3 : Fcn  Expr=u(2)*u(5)-u(1)*u(6)+u(4)*u(7)+u(3)*u(8)
  qerr4 : Fcn  Expr=-u(1)*u(5)-u(2)*u(6)-u(3)*u(7)+u(4)*u(8)
  q_ac : Outport
  wires:
  Mux1/1 -> q_ac/1
  qerr4/1 -> Mux1/4
  qerr3/1 -> Mux1/3
  qerr2/1 -> Mux1/2
  qerr1/1 -> Mux1/1
  Mux/1 -> qerr4/1, qerr3/1, qerr2/1, qerr1/1
  q_ab/1 -> Mux/2
  q_bc/1 -> Mux/1

== system collection_of_goodies/Attitude Math/axis//angle to DCM/crs matrix ==
  In1 : Inport
  Constant : Constant  Value=0
  Demux : Demux  Outputs=3
  Gain : Gain  Gain=-1  SaturateOnIntegerOverflow=on  OutDataTypeStr=Inherit: Same as input  ParamDataTypeStr=Inherit: Same as input
  Gain1 : Gain  Gain=-1  SaturateOnIntegerOverflow=on  OutDataTypeStr=Inherit: Same as input  ParamDataTypeStr=Inherit: Same as input
  Gain2 : Gain  Gain=-1  SaturateOnIntegerOverflow=on  OutDataTypeStr=Inherit: Same as input  ParamDataTypeStr=Inherit: Same as input
  Matrix Concatenation : Concatenate  NumInputs=3  Mode=Multidimensional array  ConcatenateDimension=2
  Mux : Mux  Inputs=3
  Mux1 : Mux  Inputs=3
  Mux2 : Mux  Inputs=3
  Out1 : Outport
  wires:
  In1/1 -> Demux/1
  Constant/1 -> Mux1/2, Mux/1, Mux2/3
  Demux/3 -> Mux/2, Gain1/1
  Demux/2 -> Gain/1, Mux2/1
  Gain/1 -> Mux/3
  Mux/1 -> Matrix Concatenation/1
  Gain1/1 -> Mux1/1
  Demux/1 -> Mux1/3, Gain2/1
  Mux1/1 -> Matrix Concatenation/2
  Mux2/1 -> Matrix Concatenation/3
  Gain2/1 -> Mux2/2
  Matrix Concatenation/1 -> Out1/1

== system collection_of_goodies/Attitude Math/axis//angle to DCM/crs matrix1 ==
  make : Inport
  Constant{,1..5} (6 alike) : Constant  Value=0
  Matrix Concatenation : Concatenate  NumInputs=3  Mode=Multidimensional array  ConcatenateDimension=2
  Mux : Mux  Inputs=3
  Mux1 : Mux  Inputs=3
  Mux2 : Mux  Inputs=3
  3x3 : Outport
  wires:
  make/1 -> Mux/1, Mux1/2, Mux2/3
  Mux/1 -> Matrix Concatenation/1
  Mux1/1 -> Matrix Concatenation/2
  Mux2/1 -> Matrix Concatenation/3
  Matrix Concatenation/1 -> 3x3/1
  Constant/1 -> Mux/3
  Constant1/1 -> Mux/2
  Constant2/1 -> Mux1/3
  Constant3/1 -> Mux1/1
  Constant4/1 -> Mux2/2
  Constant5/1 -> Mux2/1

== system collection_of_goodies/Attitude Math/compute attitude error/quat_multiply (relative quat) ==
  q_bc : Inport
  q_ab : Inport  Port=2
  Mux : Mux  Inputs=2
  Mux1 : Mux
  qerr1 : Fcn  Expr=u(4)*u(5)+u(3)*u(6)-u(2)*u(7)+u(1)*u(8)
  qerr2 : Fcn  Expr=-u(3)*u(5)+u(4)*u(6)+u(1)*u(7)+u(2)*u(8)
  qerr3 : Fcn  Expr=u(2)*u(5)-u(1)*u(6)+u(4)*u(7)+u(3)*u(8)
  qerr4 : Fcn  Expr=-u(1)*u(5)-u(2)*u(6)-u(3)*u(7)+u(4)*u(8)
  q_ac : Outport
  wires:
  Mux1/1 -> q_ac/1
  qerr4/1 -> Mux1/4
  qerr3/1 -> Mux1/3
  qerr2/1 -> Mux1/2
  qerr1/1 -> Mux1/1
  Mux/1 -> qerr4/1, qerr3/1, qerr2/1, qerr1/1
  q_ab/1 -> Mux/2
  q_bc/1 -> Mux/1

== system collection_of_goodies/Attitude Math/quat to DCM/Subsystem ==
  In1 : Inport
  3x3 : Reshape  OutputDimensionality=Customize  OutputDimensions=[3,3]
  Demux : Demux  Outputs=3
  Gain : Gain  Gain=-1  SaturateOnIntegerOverflow=on  OutDataTypeStr=Inherit: Same as input  ParamDataTypeStr=Inherit: Same as input
  Gain1 : Gain  Gain=-1  SaturateOnIntegerOverflow=on  OutDataTypeStr=Inherit: Same as input  ParamDataTypeStr=Inherit: Same as input
  Gain2 : Gain  Gain=-1  SaturateOnIntegerOverflow=on  OutDataTypeStr=Inherit: Same as input  ParamDataTypeStr=Inherit: Same as input
  Mux : Mux  Inputs=9
  "diag 0 " : Constant  Value=0
  Out1 : Outport
  wires:
  In1/1 -> Demux/1
  3x3/1 -> Out1/1
  "diag 0 "/1 -> Mux/1, Mux/5, Mux/9
  Mux/1 -> 3x3/1
  Demux/3 -> Mux/2, Gain1/1
  Gain/1 -> Mux/3
  Demux/2 -> Gain/1, Mux/7
  Gain1/1 -> Mux/4
  Demux/1 -> Mux/6, Gain2/1
  Gain2/1 -> Mux/8

== system collection_of_goodies/Misc/SimMechanics embedded h body/cross2 ==
  a : Inport
  b : Inport  Port=2
  Demux : Demux  Outputs=3
  Demux1 : Demux  Outputs=3
  Fcn : Fcn  Expr=-u(3)*u(5)+u(2)*u(6)
  Fcn1 : Fcn  Expr=u(3)*u(4)-u(1)*u(6)
  Fcn2 : Fcn  Expr=-u(2)*u(4)+u(1)*u(5)
  Mux : Mux  Inputs=6
  Mux1 : Mux  Inputs=3
  a x b : Outport
  wires:
  Mux/1 -> Fcn/1, Fcn1/1, Fcn2/1
  Mux1/1 -> a x b/1
  Fcn/1 -> Mux1/1
  Fcn1/1 -> Mux1/2
  Fcn2/1 -> Mux1/3
  Demux/1 -> Mux/1
  Demux/2 -> Mux/2
  Demux/3 -> Mux/3
  a/1 -> Demux/1
  Demux1/1 -> Mux/4
  Demux1/2 -> Mux/5
  Demux1/3 -> Mux/6
  b/1 -> Demux1/1

== system collection_of_goodies/Attitude Dynamics/AttitudeObserver/AttError/qconjMult ==
  q_cmd : Inport
  q_est : Inport  Port=2
  Mux : Mux  Inputs=2
  Mux1 : Mux
  qerr1 : Fcn  Expr=-u(4)*u(5)-u(3)*u(6)+u(2)*u(7)+u(1)*u(8)
  qerr2 : Fcn  Expr=u(3)*u(5)-u(4)*u(6)-u(1)*u(7)+u(2)*u(8)
  qerr3 : Fcn  Expr=-u(2)*u(5)+u(1)*u(6)-u(4)*u(7)+u(3)*u(8)
  qerr4 : Fcn  Expr=u(1)*u(5)+u(2)*u(6)+u(3)*u(7)+u(4)*u(8)
  q_err : Outport
  wires:
  q_cmd/1 -> Mux/1
  q_est/1 -> Mux/2
  Mux/1 -> qerr1/1, qerr2/1, qerr3/1, qerr4/1
  qerr1/1 -> Mux1/1
  qerr2/1 -> Mux1/2
  qerr3/1 -> Mux1/3
  qerr4/1 -> Mux1/4
  Mux1/1 -> q_err/1

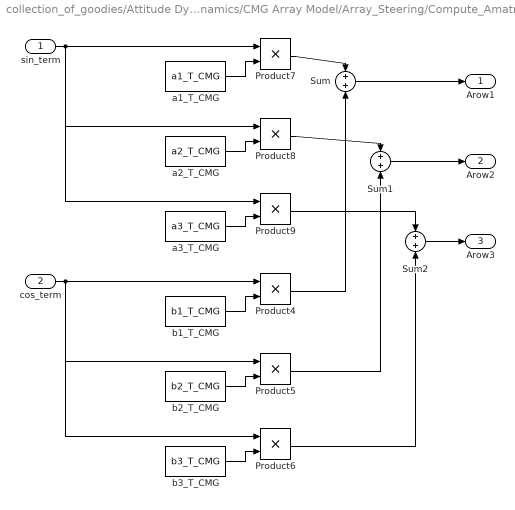
== system collection_of_goodies/Attitude Dynamics/CMG Array Model/Array_Steering/Compute_Amatrix ==
  sin_term : Inport  PortDimensions=6
  cos_term : Inport  Port=2  PortDimensions=6
  Product{4..9} (6 alike) : Product  SaturateOnIntegerOverflow=on  InputSameDT=on  OutDataTypeStr=Inherit: Same as first input
  Sum : Sum  SaturateOnIntegerOverflow=on  InputSameDT=on  OutDataTypeStr=Inherit: Same as first input
  Sum1 : Sum  SaturateOnIntegerOverflow=on  InputSameDT=on  OutDataTypeStr=Inherit: Same as first input
  Sum2 : Sum  SaturateOnIntegerOverflow=on  InputSameDT=on  OutDataTypeStr=Inherit: Same as first input
  a1_T_CMG : Constant  Value=a1_T_CMG
  a2_T_CMG : Constant  Value=a2_T_CMG
  a3_T_CMG : Constant  Value=a3_T_CMG
  b1_T_CMG : Constant  Value=b1_T_CMG
  b2_T_CMG : Constant  Value=b2_T_CMG
  b3_T_CMG : Constant  Value=b3_T_CMG
  Arow1 : Outport
  Arow2 : Outport  Port=2
  Arow3 : Outport  Port=3
  wires:
  Sum/1 -> Arow1/1
  Sum1/1 -> Arow2/1
  Sum2/1 -> Arow3/1
  Product6/1 -> Sum2/2
  Product9/1 -> Sum2/1
  Product5/1 -> Sum1/2
  Product8/1 -> Sum1/1
  Product4/1 -> Sum/2
  Product7/1 -> Sum/1
  a3_T_CMG/1 -> Product9/2
  sin_term/1 -> Product9/1, Product8/1, Product7/1
  a2_T_CMG/1 -> Product8/2
  a1_T_CMG/1 -> Product7/2
  b3_T_CMG/1 -> Product6/2
  cos_term/1 -> Product6/1, Product5/1, Product4/1
  b2_T_CMG/1 -> Product5/2
  b1_T_CMG/1 -> Product4/2

== system collection_of_goodies/Attitude Dynamics/CMG Gimbal Control System/Actuator/Bemf Phases ==
  In : Inport
  Angle : Inport  Port=2
  Elect Freq : Gain  Gain=12  SaturateOnIntegerOverflow=on  OutDataTypeStr=Inherit: Same as input  ParamDataTypeStr=Inherit: Same as input
  Mux : Mux  Inputs=2
  Product2 : Product  SaturateOnIntegerOverflow=on  InputSameDT=on  OutDataTypeStr=Inherit: Same as first input
  Product3 : Product  SaturateOnIntegerOverflow=on  InputSameDT=on  OutDataTypeStr=Inherit: Same as first input
  Trigonometric Function : Trigonometry
  Trigonometric Function1 : Trigonometry  Operator=cos
  Out : Outport  InitialOutput=0
  wires:
  Mux/1 -> Out/1
  Angle/1 -> Elect Freq/1
  In/1 -> Product2/1, Product3/1
  Trigonometric Function1/1 -> Product3/2
  Trigonometric Function/1 -> Product2/2
  Product2/1 -> Mux/1
  Product3/1 -> Mux/2
  Elect Freq/1 -> Trigonometric Function1/1, Trigonometric Function/1

== system collection_of_goodies/Attitude Dynamics/CMG Gimbal Control System/Actuator/Braking ==
  Back EMF : Inport
  Driver Voltage : Inport  Port=2
  Current : Inport  Port=3
  Terminal Voltage : Outport  InitialOutput=0
  wires:
  Driver Voltage/1 -> Terminal Voltage/1

== system collection_of_goodies/Attitude Dynamics/CMG Gimbal Control System/Actuator/Motor Coil ==
  Back EMF : Inport
  Terminal Voltage : Inport  Port=2
  Demux1 : Demux  Outputs=2
  Demux2 : Demux  Outputs=2
  Gimbal Motor Coil : TransferFcn  Denominator=[Lgm Rgm]
  Gimbal Motor Coil1 : TransferFcn  Denominator=[Lgm Rgm]
  Mux : Mux  Inputs=2
  Sum4 : Sum  Inputs=-+  SaturateOnIntegerOverflow=on  InputSameDT=on  OutDataTypeStr=Inherit: Same as first input
  Sum6 : Sum  Inputs=-+  SaturateOnIntegerOverflow=on  InputSameDT=on  OutDataTypeStr=Inherit: Same as first input
  Current : Outport  InitialOutput=0
  wires:
  Back EMF/1 -> Demux1/1
  Terminal Voltage/1 -> Demux2/1
  Sum4/1 -> Gimbal Motor Coil/1
  Sum6/1 -> Gimbal Motor Coil1/1
  Mux/1 -> Current/1
  Demux2/2 -> Sum6/2
  Demux2/1 -> Sum4/2
  Demux1/2 -> Sum6/1
  Demux1/1 -> Sum4/1
  Gimbal Motor Coil/1 -> Mux/1
  Gimbal Motor Coil1/1 -> Mux/2

== system collection_of_goodies/Attitude Dynamics/CMG Gimbal Control System/Actuator/Motor Ripple ==
  note: Ripple
      | Factor
  note: Cogging
      | Torque
      | (terms)
  Torque In : Inport
  Motor Angle : Inport  Port=2
  Amplitude : Constant  Value=rc_ampl
  Demux : Demux  Outputs=[4 5]
  Harmonic : Constant  Value=rc_harm
  Phase : Constant  Value=rc_phase
  Product : Product  SaturateOnIntegerOverflow=on  InputSameDT=on  OutDataTypeStr=Inherit: Same as first input
  Product1 : Product  SaturateOnIntegerOverflow=on  InputSameDT=on  OutDataTypeStr=Inherit: Same as first input
  Product2 : Product  SaturateOnIntegerOverflow=on  InputSameDT=on  OutDataTypeStr=Inherit: Same as first input
  Sum : Sum  Inputs=++|  SaturateOnIntegerOverflow=on  InputSameDT=on  OutDataTypeStr=Inherit: Same as first input
  Sum3 : Sum  Inputs=+  SaturateOnIntegerOverflow=on  InputSameDT=on  OutDataTypeStr=Inherit: Same as first input
  Sum4 : Sum  Inputs=+  SaturateOnIntegerOverflow=on  InputSameDT=on  OutDataTypeStr=Inherit: Same as first input
  Sum5 : Sum  SaturateOnIntegerOverflow=on  InputSameDT=on  OutDataTypeStr=Inherit: Same as first input
  Trigonometric Function : Trigonometry  Operator=cos
  Torque Ripple : Outport  InitialOutput=0
  wires:
  Product/1 -> Trigonometric Function/1
  Trigonometric Function/1 -> Product2/1
  Product2/1 -> Demux/1
  Harmonic/1 -> Product/2
  Amplitude/1 -> Product2/2
  Demux/1 -> Sum3/1
  Demux/2 -> Sum4/1
  Sum3/1 -> Sum5/1
  Sum5/1 -> Torque Ripple/1
  Product1/1 -> Sum5/2
  Sum4/1 -> Product1/1
  Torque In/1 -> Product1/2
  Motor Angle/1 -> Sum/2
  Sum/1 -> Product/1
  Phase/1 -> Sum/1

== system collection_of_goodies/Attitude Dynamics/CMG Gimbal Control System/Actuator/Torque Phases ==
  In : Inport
  Angle : Inport  Port=2
  Demux1 : Demux  Outputs=2
  Elect Freq : Gain  Gain=12  SaturateOnIntegerOverflow=on  OutDataTypeStr=Inherit: Same as input  ParamDataTypeStr=Inherit: Same as input
  Product2 : Product  SaturateOnIntegerOverflow=on  InputSameDT=on  OutDataTypeStr=Inherit: Same as first input
  Product3 : Product  SaturateOnIntegerOverflow=on  InputSameDT=on  OutDataTypeStr=Inherit: Same as first input
  Sum5 : Sum  SaturateOnIntegerOverflow=on  InputSameDT=on  OutDataTypeStr=Inherit: Same as first input
  Trigonometric Function : Trigonometry
  Trigonometric Function1 : Trigonometry  Operator=cos
  Out : Outport  InitialOutput=0
  wires:
  Elect Freq/1 -> Trigonometric Function/1, Trigonometric Function1/1
  Trigonometric Function/1 -> Product2/2
  Trigonometric Function1/1 -> Product3/2
  Angle/1 -> Elect Freq/1
  Product2/1 -> Sum5/1
  Product3/1 -> Sum5/2
  Sum5/1 -> Out/1
  Demux1/1 -> Product2/1
  Demux1/2 -> Product3/1
  In/1 -> Demux1/1

== system collection_of_goodies/Attitude Dynamics/CMG Gimbal Control System/Control/Rate Feedback ==
  Coarse/Fine : Inport
  Abs : Abs  SaturateOnIntegerOverflow=on
  Demux1 : Demux  Outputs=2
  Fine Gain Correction : Gain  Gain=1/fine  SaturateOnIntegerOverflow=on  OutDataTypeStr=Inherit: Same as input  ParamDataTypeStr=Inherit: Same as input
  Relay : Relay  OnSwitchValue=CFthreshon  OffSwitchValue=CFthreshoff
  Switch : Switch  Threshold=.5  SaturateOnIntegerOverflow=on  InputSameDT=on
  Composite : Outport  InitialOutput=0
  wires:
  Coarse/Fine/1 -> Demux1/1
  Demux1/2 -> Fine Gain Correction/1
  Fine Gain Correction/1 -> Switch/3
  Relay/1 -> Switch/2
  Demux1/1 -> Switch/1, Abs/1
  Abs/1 -> Relay/1
  Switch/1 -> Composite/1

== system collection_of_goodies/Attitude Dynamics/CMG Gimbal Control System/Control/Rate Loop Compensation ==
  Rate Error : Inport
  "\"Bi-Quad\"" : TransferFcn  Numerator=filt1n  Denominator=filt1d
  Integrator : Integrator  LimitOutput=on  UpperSaturationLimit=Isat  LowerSaturationLimit=-Isat
  Lead/Lag : TransferFcn  Numerator=filt2n  Denominator=filt2d
  Current Cmd : Outport  InitialOutput=0
  wires:
  "\"Bi-Quad\""/1 -> Lead/Lag/1
  Rate Error/1 -> "\"Bi-Quad\""/1
  Integrator/1 -> Current Cmd/1
  Lead/Lag/1 -> Integrator/1

== system collection_of_goodies/Attitude Dynamics/CMG Gimbal Control System/Control/Resolver Logic ==
  Resolver : Inport
  Demux1 : Demux
  Gain1 : Gain  Gain=1/32  SaturateOnIntegerOverflow=on  OutDataTypeStr=Inherit: Same as input  ParamDataTypeStr=Inherit: Same as input
  Trigonometric Function : Trigonometry  Operator=atan2
  Trigonometric Function1 : Trigonometry  Operator=atan2
  Measured Shaft Angle : Outport  InitialOutput=0
  wires:
  Resolver/1 -> Demux1/1
  Demux1/1 -> Trigonometric Function/1
  Demux1/2 -> Trigonometric Function/2
  Demux1/3 -> Trigonometric Function1/1
  Demux1/4 -> Trigonometric Function1/2
  Trigonometric Function1/1 -> Measured Shaft Angle/1
  Trigonometric Function/1 -> Gain1/1

== system collection_of_goodies/Attitude Dynamics/CMG Gimbal Control System/Control/SpeedQuant ==
  note: Qspeed in sec/rad to emulate timing of one rev
  In : Inport
  Math Function : Math  Operator=reciprocal  SaturateOnIntegerOverflow=on
  Math Function1 : Math  Operator=reciprocal  SaturateOnIntegerOverflow=on
  Qspeed : Quantizer  QuantizationInterval=Qspeed
  SpeedMin : Saturate  UpperLimit=inf  LowerLimit=Smin
  Out : Outport  InitialOutput=0
  wires:
  Math Function/1 -> Qspeed/1
  Math Function1/1 -> Out/1
  Qspeed/1 -> Math Function1/1
  In/1 -> SpeedMin/1
  SpeedMin/1 -> Math Function/1

== system collection_of_goodies/Attitude Dynamics/CMG Gimbal Control System/Control/Spin Loop Compensation ==
  Rate Error : Inport
  Integrator : Integrator  InitialCondition=spin_init  LimitOutput=on  UpperSaturationLimit=IsatSp  LowerSaturationLimit=-IsatSp
  Lead/Lag : TransferFcn  Numerator=filts2n  Denominator=filts2d
  filts1n : Gain  Gain=filts1n  SaturateOnIntegerOverflow=on  OutDataTypeStr=Inherit: Same as input  ParamDataTypeStr=Inherit: Same as input
  Current Cmd : Outport  InitialOutput=0
  wires:
  Rate Error/1 -> Lead/Lag/1
  Lead/Lag/1 -> filts1n/1
  filts1n/1 -> Integrator/1
  Integrator/1 -> Current Cmd/1

== system collection_of_goodies/Attitude Dynamics/CMG Gimbal Control System/Control/TorqueComm ==
  Current Command : Inport
  Meas Shaft Angle : Inport  Port=2
  Gain1 : Gain  Gain=12  SaturateOnIntegerOverflow=on  OutDataTypeStr=Inherit: Same as input  ParamDataTypeStr=Inherit: Same as input
  Mux : Mux  Inputs=2
  Product : Product  SaturateOnIntegerOverflow=on  InputSameDT=on  OutDataTypeStr=Inherit: Same as first input
  Product1 : Product  SaturateOnIntegerOverflow=on  InputSameDT=on  OutDataTypeStr=Inherit: Same as first input
  Trigonometric Function : Trigonometry
  Trigonometric Function1 : Trigonometry  Operator=cos
  Current Cmds : Outport  InitialOutput=0
  wires:
  Mux/1 -> Current Cmds/1
  Current Command/1 -> Product/1, Product1/1
  Meas Shaft Angle/1 -> Gain1/1
  Gain1/1 -> Trigonometric Function/1, Trigonometric Function1/1
  Trigonometric Function/1 -> Product/2
  Trigonometric Function1/1 -> Product1/2
  Product/1 -> Mux/1
  Product1/1 -> Mux/2

== system collection_of_goodies/Attitude Dynamics/CMG Gimbal Control System/Drive/Current Loop 1 ==
  CurrentCmd : Inport
  Current : Inport  Port=2
  AAF : TransferFcn  Denominator=IgmAAFd
  Current Loop Compensation : TransferFcn  Numerator=Igm1n  Denominator=Igm1d
  PWM : Gain  SaturateOnIntegerOverflow=on  OutDataTypeStr=Inherit: Same as input  ParamDataTypeStr=Inherit: Same as input
  Sum : Sum  Inputs=+-  SaturateOnIntegerOverflow=on  InputSameDT=on  OutDataTypeStr=Inherit: Same as first input
  Vbus : Saturate  UpperLimit=Vsat  LowerLimit=-Vsat
  VcoilQuant : Quantizer  QuantizationInterval=Qvcoil
  Vanalog : Outport  InitialOutput=0
  CurSense : Outport  Port=2  InitialOutput=0
  wires:
  CurrentCmd/1 -> Sum/1
  VcoilQuant/1 -> Vanalog/1
  Vbus/1 -> VcoilQuant/1
  Current/1 -> AAF/1
  PWM/1 -> Vbus/1
  Current Loop Compensation/1 -> PWM/1
  AAF/1 -> Sum/2, CurSense/1
  Sum/1 -> Current Loop Compensation/1

== system collection_of_goodies/Attitude Dynamics/CMG Gimbal Control System/Drive/Current Loop 2 ==
  CurrentCmd : Inport
  Current : Inport  Port=2
  AAF : TransferFcn  Denominator=IgmAAFd
  Current Loop Compensation : TransferFcn  Numerator=Igm1n  Denominator=Igm1d
  PWM : Gain  SaturateOnIntegerOverflow=on  OutDataTypeStr=Inherit: Same as input  ParamDataTypeStr=Inherit: Same as input
  Sum : Sum  Inputs=+-  SaturateOnIntegerOverflow=on  InputSameDT=on  OutDataTypeStr=Inherit: Same as first input
  Vbus : Saturate  UpperLimit=Vsat  LowerLimit=-Vsat
  VcoilQuant : Quantizer  QuantizationInterval=Qvcoil
  Vanalog : Outport  InitialOutput=0
  CurSense : Outport  Port=2  InitialOutput=0
  wires:
  Sum/1 -> Current Loop Compensation/1
  AAF/1 -> CurSense/1, Sum/2
  Current Loop Compensation/1 -> PWM/1
  PWM/1 -> Vbus/1
  Current/1 -> AAF/1
  Vbus/1 -> VcoilQuant/1
  VcoilQuant/1 -> Vanalog/1
  CurrentCmd/1 -> Sum/1

== system collection_of_goodies/Attitude Dynamics/CMG Gimbal Control System/Sensor/Resolvers ==
  Truth Angle : Inport
  32x : Gain  Gain=32  SaturateOnIntegerOverflow=on  OutDataTypeStr=Inherit: Same as input  ParamDataTypeStr=Inherit: Same as input
  AAF{,1..3} (4 alike) : TransferFcn  Denominator=[1/(2*pi*250) 1]
  Mux4 : Mux
  Trigonometric Function : Trigonometry
  Trigonometric Function1 : Trigonometry  Operator=cos
  Trigonometric Function2 : Trigonometry
  Trigonometric Function3 : Trigonometry  Operator=cos
  Resolver Out : Outport  InitialOutput=0
  wires:
  Mux4/1 -> Resolver Out/1
  AAF/1 -> Mux4/1
  Trigonometric Function/1 -> AAF/1
  32x/1 -> Trigonometric Function/1, Trigonometric Function1/1
  Truth Angle/1 -> 32x/1, Trigonometric Function2/1, Trigonometric Function3/1
  Trigonometric Function1/1 -> AAF1/1
  Trigonometric Function2/1 -> AAF2/1
  Trigonometric Function3/1 -> AAF3/1
  AAF1/1 -> Mux4/2
  AAF2/1 -> Mux4/3
  AAF3/1 -> Mux4/4
